simulink model "ex6imppdco"  (R2025b)
settings: Solver=VariableStepAuto  StartTime=0.0  StopTime=396  RelTol=1e-3
values from neighbouring files (symbols this model uses):
  IJ = inv(J)    [ex13.m]    (also in ex6.m)
  J = jacobian(f,[x1,x2])    [ex1.m]    (also in ex13.m = diag([10400, 8200, 9200]); ex2.m; ex6.m = diag([7000,5900,9600]))
  q0 = [0.68438, -0.56827,-0.10002,-0.44574]'    [ex13.m]    (also in ex6.m = [1;0;0;0])
  qr = [-0.068456;-.55729;0.82576;-0.053478]    [ex6.m]
  w0 = [0;0;0]    [ex13.m]    (also in ex6.m)
libraries: vrlib x1
settings Model: Creator=Esteban  LastModifiedBy=Esteban

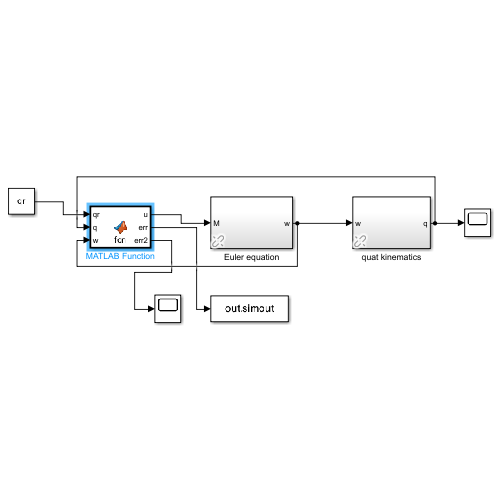
[thumbnail: Simulink's stored preview of the top-level diagram]
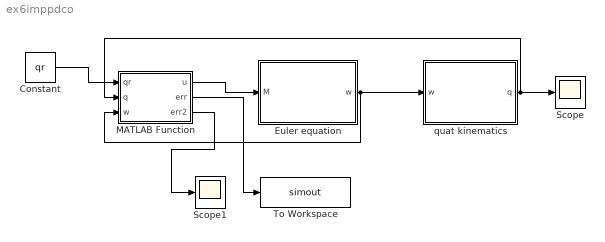
== system ex6imppdco ==
  Constant : Constant  Value=qr
  Euler equation : Subsystem  AncestorBlock=lib_rotations_2014/Euler equation
  MATLAB Function : MATLAB Function  TreatAsAtomicUnit=on
  Scope : Scope
  Scope1 : Scope
      settings: ActiveDisplayYMinimum=-3.8907250150837633  ActiveDisplayYMaximum=40.576165895097205
  To Workspace : ToWorkspace  VariableName=simout  SaveFormat=Timeseries  SampleTime=-1
  quat kinematics : Subsystem  AncestorBlock=lib_rotations_2014/quat kinematics
  wires:
  MATLAB Function/1(u) -> Euler equation/1(M)
  Euler equation/1(w) -> MATLAB Function/3(w), quat kinematics/1(w)
  quat kinematics/1(q) -> MATLAB Function/2(q), Scope/1
  MATLAB Function/3(err2) -> Scope1/1
  MATLAB Function/2(err) -> To Workspace/1
  Constant/1 -> MATLAB Function/1(qr)

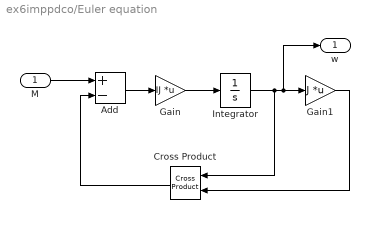
== system ex6imppdco/Euler equation ==
  M : Inport
  Add : Sum  Inputs=+-
  Cross Product : vrlib/Utilities/Cross Product
  Gain : Gain  Gain=IJ  Multiplication=Matrix(K*u)
  Gain1 : Gain  Gain=J  Multiplication=Matrix(K*u)
  Integrator : Integrator  InitialCondition=w0
  w : Outport  VectorParamsAs1DForOutWhenUnconnected=off
  wires:
  Cross Product/1 -> Add/2
  Add/1 -> Gain/1
  Gain1/1 -> Cross Product/2
  Gain/1 -> Integrator/1
  Integrator/1 -> Gain1/1, w/1, Cross Product/1
  M/1 -> Add/1

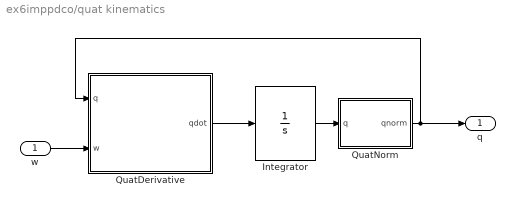
== system ex6imppdco/quat kinematics ==
  w : Inport  PortDimensions=3
  Integrator : Integrator  InitialCondition=q0
  QuatDerivative : MATLAB Function  TreatAsAtomicUnit=on
  QuatNorm : MATLAB Function  TreatAsAtomicUnit=on
  q : Outport  PortDimensions=4  VectorParamsAs1DForOutWhenUnconnected=off
  wires:
  w/1 -> QuatDerivative/2(w)
  QuatDerivative/1(qdot) -> Integrator/1
  QuatNorm/1(qnorm) -> QuatDerivative/1(q), q/1
  Integrator/1 -> QuatNorm/1(q)

== matlab function ex6imppdco/quat kinematics/QuatDerivative ==
  data: q input; qdot output; w input
function qdot= QuatDerivative(q,w)
%#codegen
omegaq=[0; w];
Q=[q(1) -q(2) -q(3) -q(4);
    q(2) q(1) -q(4) q(3);
    q(3) q(4) q(1) -q(2);
    q(4) -q(3) q(2) q(1)];
qdot=Q*omegaq/2;

== matlab function ex6imppdco/quat kinematics/QuatNorm ==
  data: q input; qnorm output
function qnorm = QuatNorm(q)
%#codegen
qnorm=zeros(4,1);
q2=sqrt(q'*q);
qnorm=q/q2;

== matlab function ex6imppdco/MATLAB Function ==
  data: qr input; u output; q input; w input; err output; err2 output
function [u,err,err2] = fcn(qr,q,w)

k1 = 22;
k2 = 196;

qs = [q(1);-q(2:4)];

dq = quatprod(qs,qr);

err = norm(dq(2:4));

u = k1*dq(2:4)-k2*w;

err2 = norm(u);
